simulink model "model_ciagly_dodatkowy"  (R2020a)
settings: Solver=VariableStepAuto  StartTime=0.0  StopTime=10.0  RelTol=1e-3
settings Model: Creator=jakub  LastModifiedBy=jakub

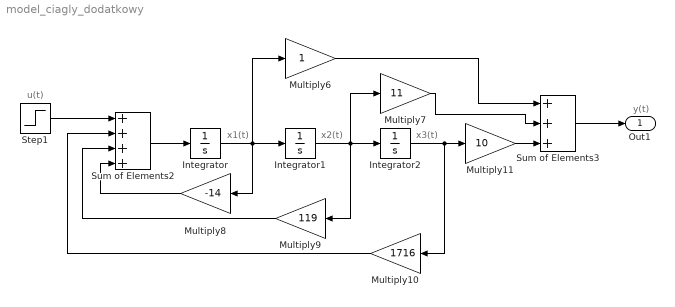
== system model_ciagly_dodatkowy ==
  note: x1(t)
  note: x3(t)
  note: x2(t)
  note: u(t)
  note: y(t)
  Integrator : Integrator
  Integrator1 : Integrator
  Integrator2 : Integrator
  Multiply10 : Gain  Gain=1716
  Multiply11 : Gain  Gain=10
  Multiply6 : Gain
  Multiply7 : Gain  Gain=11
  Multiply8 : Gain  Gain=-14
  Multiply9 : Gain  Gain=119
  Step1 : Step  SampleTime=0
  Sum of Elements2 : Sum  Inputs=++++
  Sum of Elements3 : Sum  Inputs=+++
  Out1 : Outport
  wires:
  Multiply11/1 -> Sum of Elements3/3
  Integrator1/1 -> Integrator2/1, Multiply7/1, Multiply9/1
  Step1/1 -> Sum of Elements2/1
  Sum of Elements3/1 -> Out1/1
  Multiply6/1 -> Sum of Elements3/1
  Multiply8/1 -> Sum of Elements2/4
  Multiply10/1 -> Sum of Elements2/2
  Integrator/1 -> Integrator1/1, Multiply8/1, Multiply6/1
  Sum of Elements2/1 -> Integrator/1
  Multiply9/1 -> Sum of Elements2/3
  Integrator2/1 -> Multiply10/1, Multiply11/1
  Multiply7/1 -> Sum of Elements3/2
